simulink model "control_model_new_2018a"  (R2018b)
settings: Solver=VariableStepAuto  StartTime=0.0  StopTime=100  RelTol=1e-04
libraries: simulink x2
settings Model: Creator=geraldlow  LastModifiedBy=geraldlow

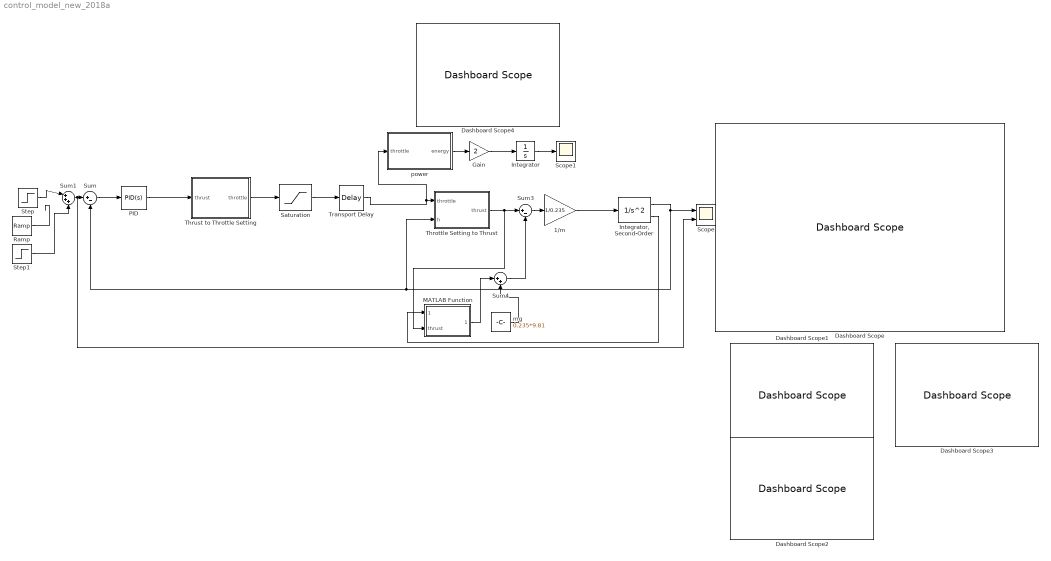
== system control_model_new_2018a ==
  1/m : Gain  Gain=1/0.235
  Dashboard Scope : DashboardScope  WebBlockId=85
  Dashboard Scope1 : DashboardScope  WebBlockId=86
  Dashboard Scope2 : DashboardScope  WebBlockId=87
  Dashboard Scope3 : DashboardScope  WebBlockId=89
  Dashboard Scope4 : DashboardScope  WebBlockId=88
  Gain : Gain  Gain=2
  Integrator : Integrator
  "Integrator, Second-Order" : SecondOrderIntegrator  ICX=0  LimitX=on  LowerLimitX=0
  MATLAB Function : MATLAB Function  TreatAsAtomicUnit=on
  PID : simulink/Continuous/PID Controller  Controller=PID  Form=Parallel  TimeDomain=Continuous-time  SampleTime=-1  IntegratorMethod=Forward Euler  FilterMethod=Forward Euler  ControllerParametersSource=internal  P=.2  I=1.3e-01  D=1.8  UseFilter=on  N=78.67  TunerSelectOption=Transfer Function Based (PID Tuner App)  InitialConditionSource=internal  InitialConditionForIntegrator=0  InitialConditionForFilter=0  DifferentiatorICPrevScaledInput=0  ExternalReset=none  TrackingMode=off  Kt=1  LimitOutput=off  UpperSaturationLimit=inf  LowerSaturationLimit=-inf  LinearizeAsGain=on  AntiWindupMode=none  Kb=1  POutMin=[]  POutMax=[]  IOutMin=[]  IOutMax=[]  DOutMin=[]  DOutMax=[]  NOutMin=[]  NOutMax=[]  SumOutMin=[]  SumOutMax=[]  SaturationOutMin=[]  SaturationOutMax=[]  PParamMin=[]  PParamMax=[]  IParamMin=[]  IParamMax=[]  DParamMin=[]  DParamMax=[]  NParamMin=[]  NParamMax=[]  KbParamMin=[]  KbParamMax=[]  KtParamMin=[]  KtParamMax=[]  KbOutMin=[]  KbOutMax=[]  KtOutMin=[]  KtOutMax=[]  IntegratorOutMin=[]  IntegratorOutMax=[]  FilterOutMin=[]  FilterOutMax=[]  SumI1OutMin=[]  SumI1OutMax=[]  SumI2OutMin=[]  SumI2OutMax=[]  SumI3OutMin=[]  SumI3OutMax=[]  SumI4OutMin=[]  SumI4OutMax=[]  SumDOutMin=[]  SumDOutMax=[]  DifferentiatorOutMin=[]  DifferentiatorOutMax=[]  FilterDiffOutCoefMin=[]  FilterDiffOutCoefMax=[]  ReciprocalOutMin=[]  ReciprocalOutMax=[]  SumDenOutMin=[]  SumDenOutMax=[]  SumNumOutMin=[]  SumNumOutMax=[]  DivideOutMin=[]  DivideOutMax=[]  IntegratorContinuousStateAttributes=''  IntegratorStateMustResolveToSignalObject=off  IntegratorRTWStateStorageClass=Auto  FilterContinuousStateAttributes=''  FilterStateMustResolveToSignalObject=off  FilterRTWStateStorageClass=Auto  ParallelPVariant=InternalParameters  IdealPVariant=Disabled  IVariant=InternalParameters  DVariant=InternalParameters  IntegratorVariant=Continuous  SatVariant=Disabled  AWVariant=Passthrough  PCopyVariant=Disabled  TRVariant=Disabled  FdbkBlocksVariant=Forward  IdealPFdbkVariant=Disabled  SatFdbkVariant=Disabled  DerivativeFilterVariant=ContFilter  NVariant=InternalParameters  NCopyVariant=Disabled  FilterICVariant=InternalICsFilter  IntegratorICVariant=InternalICs  ExternalResetVariant=Disabled  TRSumVariant=Passthrough  SumFdbkVariant=Disabled  SumVariant=Sum_PID
  Ramp : simulink/Sources/Ramp  slope=.125  start=15  InitialOutput=0
  Saturation : Saturate  UpperLimit=100  LowerLimit=0
  Scope : Scope  NumInputPorts=2
  Scope1 : Scope
  Step : Step  Time=10  After=.7  SampleTime=0
  Step1 : Step  Time=20  After=.5  SampleTime=0
  Sum : Sum  Inputs=|+-
  Sum1 : Sum  Inputs=|+++
  Sum3 : Sum  Inputs=|+-
  Sum4 : Sum  Inputs=|++
  Throttle Setting to Thrust : MATLAB Function  TreatAsAtomicUnit=on
  Thrust to Throttle Setting : MATLAB Function  TreatAsAtomicUnit=on
  Transport Delay : TransportDelay  DelayTime=.2
  mg : Constant  Value=0.235*9.81
  power : MATLAB Function  TreatAsAtomicUnit=on
  wires:
  Sum/1 -> PID/1
  Thrust to Throttle Setting/1(throttle) -> Saturation/1
  mg/1 -> Sum4/2
  Sum3/1 -> 1/m/1
  "Integrator, Second-Order"/1 -> Scope/1, Sum/2, Throttle Setting to Thrust/2(h)
  Sum1/1 -> Sum/1, Scope/2
  Sum4/1 -> Sum3/2
  MATLAB Function/1(friction) -> Sum4/1
  Throttle Setting to Thrust/1(thrust) -> MATLAB Function/2(thrust), Sum3/1
  1/m/1 -> "Integrator, Second-Order"/1
  Ramp/1 -> ?
  PID/1 -> Thrust to Throttle Setting/1(thrust)
  Step/1 -> Sum1/1
  Step1/1 -> Sum1/3
  Integrator/1 -> Scope1/1
  power/1(energy) -> Gain/1
  Gain/1 -> Integrator/1
  "Integrator, Second-Order"/2 -> MATLAB Function/1(velocity)
  Saturation/1 -> Transport Delay/1
  Transport Delay/1 -> Throttle Setting to Thrust/1(throttle), power/1(throttle)

== matlab function control_model_new_2018a/Throttle Setting to Thrust ==
  data: throttle input; thrust output; h input
function thrust = fcn(throttle, h)
r=0.1524;
if throttle < 1
   thrust = 0;
elseif throttle > 88
   thrust=2*9.81*.66;
else
   thrust=2*9.81*(0.1+(.66-0.1)/(88-1)*(throttle-1));
end

   h=h+0.05;
   thrust=thrust/(1-r^2/(16*h^2))-h*r^2/(2*sqrt(4*h^2)^3);
end

== matlab function control_model_new_2018a/Thrust to Throttle Setting ==
  data: thrust input; throttle output
function throttle = fcn(thrust)
% (.66-0.1)/(88-1)*2*9.81 = 0.1263
throttle = (thrust / 0.1263)+.8;
end

== matlab function control_model_new_2018a/MATLAB Function ==
  data: velocity input; friction output; thrust input
function friction   = fcn(velocity, thrust)
epsilon = 0.005; %small perturbation
mg = 0.235*9.81;
% Get reasonable values for x1, x2, l
x1 = 0.0125;
x2 = 0.0125;
l = 0.221;
netforce = thrust-mg; %mg should be a constant defined.
mu = 0.15; %coeff of dynamic friction
%static friction
if abs(velocity) < epsilon && abs(netforce) < 0.13*9.81 && netforce > 0
    friction = netforce;
elseif abs(velocity) < epsilon && abs(netforce) < 0.13*9.81 && netforce < 0
    friction = -netforce;
elseif velocity > 0
    friction=2*mu*(mg*x1-thrust*x2)/l;
elseif velocity < 0
    friction=-2*mu*(mg*x1-thrust*x2)/l;
else
    friction=0;
end

== matlab function control_model_new_2018a/power ==
  data: throttle input; energy output
function energy =power(throttle)
epsilon=0.001;
if throttle<epsilon
    energy=0;
elseif throttle<90

energy=(500-10)/90*throttle+10;
else
    energy=200;
end
end
